simulink model "OptoShield_InputsOutputs"  (R2018b)
settings: Solver=FixedStepDiscrete  StartTime=0.0  StopTime=inf  FixedStep=0.010  RelTol=1e-3  EnableMultiTasking=on
libraries: Opto x4
settings Model: SimulationMode=external  ExtModeTrigDuration=2  Creator=Gergely  LastModifiedBy=Gergely
settings OptimizationCC: EnhancedBackFolding=on  PassReuseOutputArgsAs=Individual arguments  MaxStackSize=64  OptimizeBlockOrder=speed  DifferentSizesBufferReuse=on  OptimizationCustomize=off
settings DebuggingCC: ParameterTunabilityLossMsg=error  LibraryContextMissingDiagnostic=none
settings HardwareCC: ProdBitPerInt=16  ProdBitPerPointer=16  ProdBitPerSizeT=16  ProdBitPerPtrDiffT=16  ProdLargestAtomicFloat=None  ProdWordSize=8  ProdHWDeviceType=Atmel->AVR
settings SFSimCC: SimUseLocalCustomCode=off  MATLABDynamicMemAlloc=off
settings RTWCC: SystemTargetFile=ert.tlc  HardwareBoard=Arduino Uno  TemplateMakefile=ert_default_tmf  GenerateReport=on  RTWUseLocalCustomCode=off  Toolchain=Arduino AVR  BuildConfiguration=Faster Runs  IncludeHyperlinkInReport=on  LaunchReport=on  GenerateTraceInfo=on  GenerateTraceReport=on  GenerateTraceReportSl=on  GenerateTraceReportSf=on  GenerateTraceReportEml=on
settings CodeAppCC: ForceParamTrailComments=on  IgnoreCustomStorageClasses=off  OperatorAnnotations=on  SimulinkDataObjDesc=on  SFDataObjDesc=on  InsertBlockDesc=on
settings ERTTargetCC: SupportContinuousTime=on  SupportVariableSizeSignals=on

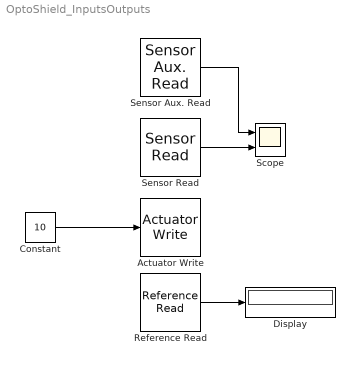
== system OptoShield_InputsOutputs ==
  Actuator Write : Opto/Actuator Write
      settings: SourceProductName=AutomationShield
  Constant : Constant  Value=10
  Display : Display
  Reference Read : Opto/Reference Read  ReadoutRadio=Percentage  Ts=0.01
      settings: SourceProductName=AutomationShield
  "Scope " : Scope  NumInputPorts=2
  Sensor Aux. Read : Opto/Sensor Aux. Read  ReadoutRadio=Voltage  Ts=0.01
      settings: SourceProductName=AutomationShield
  Sensor Read : Opto/Sensor Read  ReadoutRadio=Voltage  MaxLDR=860  Parameter3=0.01
      settings: SourceProductName=AutomationShield
  wires:
  Sensor Read/1 -> "Scope "/2
  Constant/1 -> Actuator Write/1
  Sensor Aux. Read/1 -> "Scope "/1
  Reference Read/1 -> Display/1
